simulink model "Gear"  (R2021b)
settings: Solver=VariableStepAuto  StartTime=0.0  StopTime=10.0  RelTol=1e-3
settings Model: Creator=david  LastModifiedBy=david

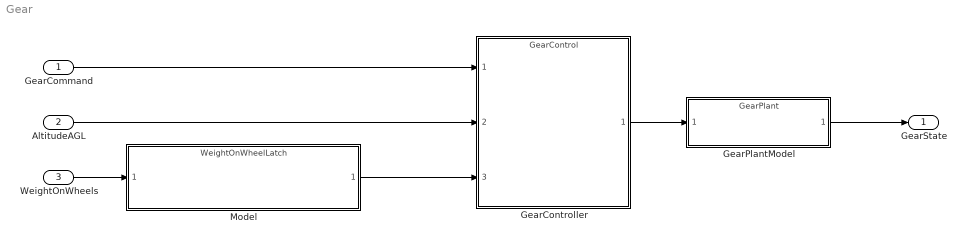
== system Gear ==
  GearCommand : Inport  OutDataTypeStr=Enum: GearCommandEnum
  AltitudeAGL : Inport  Port=2
  WeightOnWheels : Inport  Port=3
  GearController : ModelReference  ModelNameDialog=GearControl.mdl  SimulationMode=Normal  ModelReferenceVersion=1.40
  GearPlantModel : ModelReference  ModelNameDialog=GearPlant  SimulationMode=Normal  ModelReferenceVersion=1.9
  Model : ModelReference  ModelNameDialog=WeightOnWheelLatch.mdl  SimulationMode=Normal  ModelReferenceVersion=1.1
  GearState : Outport  OutDataTypeStr=Enum: GearStateEnum
  wires:
  GearCommand/1 -> GearController/1
  AltitudeAGL/1 -> GearController/2
  GearController/1 -> GearPlantModel/1
  GearPlantModel/1 -> GearState/1
  WeightOnWheels/1 -> Model/1
  Model/1 -> GearController/3
